simulink model "ACC_CC_model_4_15"  (R2018b)
settings: Solver=FixedStepAuto  StartTime=0.0  StopTime=20  RelTol=1e-3
InitFcn:
  | step=0.001;%时间步长
  | 
  | 
  | run parma2.m
libraries: simulink x2, Solver_SF x1, fuzblock x1
settings Model: Creator=Administrator  LastModifiedBy=61602
settings SFSimCC: SimUseLocalCustomCode=off
settings RTWCC: RTWUseLocalCustomCode=off

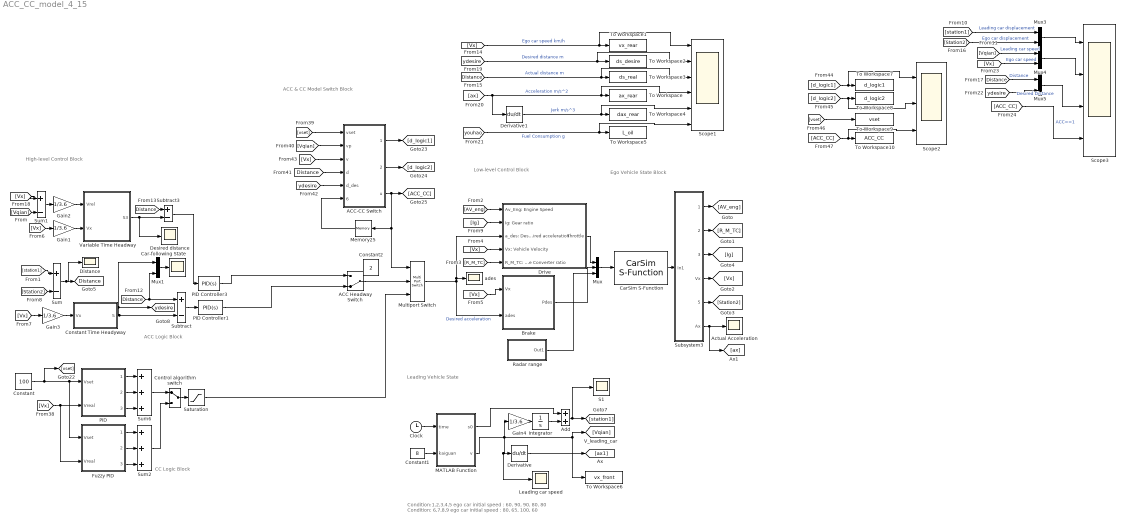
== system ACC_CC_model_4_15 ==
  note: Condition:1,2,3,4,5 ego car initial speed：60, 90, 90, 80, 80
      | Condition: 6,7,8,9   ego car initial speed：80, 65, 100, 60
  note: Leading Vehicle State
  note: ACC & CC Model
      | Switch Block
  note: High-level Control Block
  note: ACC Logic Block
  note: CC Logic Block
  note: Low-level
      | Control Block
  note: Ego Vehicle State
      | Block
  ACC Headway Switch : ManualSwitch  CurrentSetting=0
  ACC-CC Switch : MATLAB Function  TreatAsAtomicUnit=on
  Actual Acceleration : Scope
  Add : Sum
  Brake : Subsystem
  Car-following State : Scope
  "CarSim S-Function " : Solver_SF/CarSim S-Function  Priority=1  SIMFILE=simfile.sim
  Clock : Clock
  Constant : Constant  Value=100
  Constant Time Headyway : Subsystem
  Constant1 : Constant  Value=8
  Constant2 : Constant  Value=2
  Control algorithm switch : ManualSwitch
  Derivative : Derivative
  Derivative1 : Derivative
  "Desired distance " : Scope
  Distance : Scope
  Drive : Subsystem
  Fuzzy PID : Subsystem
  Gain{1..4} (4 alike) : Gain  Gain=1/3.6
  Integrator : Integrator
  Leading car speed : Scope
  MATLAB Function : MATLAB Function  TreatAsAtomicUnit=on
  Memory25 : Memory
  Multiport Switch : MultiPortSwitch  Inputs=2
  Mux : Mux  Inputs=3
  Mux{1,3..5} (4 alike) : Mux  Inputs=2
  PID : Subsystem
  PID Controller1 : simulink/Continuous/PID Controller  Controller=PID  Form=Parallel  TimeDomain=Continuous-time  SampleTime=-1  IntegratorMethod=Forward Euler  FilterMethod=Forward Euler  ControllerParametersSource=internal  P=4  I=0.01  D=2  UseFilter=on  N=100  TunerSelectOption=Transfer Function Based (PID Tuner App)  InitialConditionSource=internal  InitialConditionForIntegrator=0  InitialConditionForFilter=0  DifferentiatorICPrevScaledInput=0  ExternalReset=none  TrackingMode=off  Kt=1  LimitOutput=off  UpperSaturationLimit=inf  LowerSaturationLimit=-inf  LinearizeAsGain=on  AntiWindupMode=none  Kb=1  POutMin=[]  POutMax=[]  IOutMin=[]  IOutMax=[]  DOutMin=[]  DOutMax=[]  NOutMin=[]  NOutMax=[]  SumOutMin=[]  SumOutMax=[]  SaturationOutMin=[]  SaturationOutMax=[]  PParamMin=[]  PParamMax=[]  IParamMin=[]  IParamMax=[]  DParamMin=[]  DParamMax=[]  NParamMin=[]  NParamMax=[]  KbParamMin=[]  KbParamMax=[]  KtParamMin=[]  KtParamMax=[]  KbOutMin=[]  KbOutMax=[]  KtOutMin=[]  KtOutMax=[]  IntegratorOutMin=[]  IntegratorOutMax=[]  FilterOutMin=[]  FilterOutMax=[]  SumI1OutMin=[]  SumI1OutMax=[]  SumI2OutMin=[]  SumI2OutMax=[]  SumI3OutMin=[]  SumI3OutMax=[]  SumI4OutMin=[]  SumI4OutMax=[]  SumDOutMin=[]  SumDOutMax=[]  DifferentiatorOutMin=[]  DifferentiatorOutMax=[]  FilterDiffOutCoefMin=[]  FilterDiffOutCoefMax=[]  ReciprocalOutMin=[]  ReciprocalOutMax=[]  SumDenOutMin=[]  SumDenOutMax=[]  SumNumOutMin=[]  SumNumOutMax=[]  DivideOutMin=[]  DivideOutMax=[]  IntegratorContinuousStateAttributes=''  IntegratorStateMustResolveToSignalObject=off  IntegratorRTWStateStorageClass=Auto  FilterContinuousStateAttributes=''  FilterStateMustResolveToSignalObject=off  FilterRTWStateStorageClass=Auto  ParallelPVariant=InternalParameters  IdealPVariant=Disabled  IVariant=InternalParameters  DVariant=InternalParameters  IntegratorVariant=Continuous  SatVariant=Disabled  AWVariant=Passthrough  PCopyVariant=Disabled  TRVariant=Disabled  FdbkBlocksVariant=Forward  IdealPFdbkVariant=Disabled  SatFdbkVariant=Disabled  DerivativeFilterVariant=ContFilter  NVariant=InternalParameters  NCopyVariant=Disabled  FilterICVariant=InternalICsFilter  IntegratorICVariant=InternalICs  ExternalResetVariant=Disabled  TRSumVariant=Passthrough  SumFdbkVariant=Disabled  SumVariant=Sum_PID
  PID Controller3 : simulink/Continuous/PID Controller  Controller=PID  Form=Parallel  TimeDomain=Continuous-time  SampleTime=-1  IntegratorMethod=Forward Euler  FilterMethod=Forward Euler  ControllerParametersSource=internal  P=4  I=0.01  D=2  UseFilter=on  N=100  TunerSelectOption=Transfer Function Based (PID Tuner App)  InitialConditionSource=internal  InitialConditionForIntegrator=0  InitialConditionForFilter=0  DifferentiatorICPrevScaledInput=0  ExternalReset=none  TrackingMode=off  Kt=1  LimitOutput=off  UpperSaturationLimit=inf  LowerSaturationLimit=-inf  LinearizeAsGain=on  AntiWindupMode=none  Kb=1  POutMin=[]  POutMax=[]  IOutMin=[]  IOutMax=[]  DOutMin=[]  DOutMax=[]  NOutMin=[]  NOutMax=[]  SumOutMin=[]  SumOutMax=[]  SaturationOutMin=[]  SaturationOutMax=[]  PParamMin=[]  PParamMax=[]  IParamMin=[]  IParamMax=[]  DParamMin=[]  DParamMax=[]  NParamMin=[]  NParamMax=[]  KbParamMin=[]  KbParamMax=[]  KtParamMin=[]  KtParamMax=[]  KbOutMin=[]  KbOutMax=[]  KtOutMin=[]  KtOutMax=[]  IntegratorOutMin=[]  IntegratorOutMax=[]  FilterOutMin=[]  FilterOutMax=[]  SumI1OutMin=[]  SumI1OutMax=[]  SumI2OutMin=[]  SumI2OutMax=[]  SumI3OutMin=[]  SumI3OutMax=[]  SumI4OutMin=[]  SumI4OutMax=[]  SumDOutMin=[]  SumDOutMax=[]  DifferentiatorOutMin=[]  DifferentiatorOutMax=[]  FilterDiffOutCoefMin=[]  FilterDiffOutCoefMax=[]  ReciprocalOutMin=[]  ReciprocalOutMax=[]  SumDenOutMin=[]  SumDenOutMax=[]  SumNumOutMin=[]  SumNumOutMax=[]  DivideOutMin=[]  DivideOutMax=[]  IntegratorContinuousStateAttributes=''  IntegratorStateMustResolveToSignalObject=off  IntegratorRTWStateStorageClass=Auto  FilterContinuousStateAttributes=''  FilterStateMustResolveToSignalObject=off  FilterRTWStateStorageClass=Auto  ParallelPVariant=InternalParameters  IdealPVariant=Disabled  IVariant=InternalParameters  DVariant=InternalParameters  IntegratorVariant=Continuous  SatVariant=Disabled  AWVariant=Passthrough  PCopyVariant=Disabled  TRVariant=Disabled  FdbkBlocksVariant=Forward  IdealPFdbkVariant=Disabled  SatFdbkVariant=Disabled  DerivativeFilterVariant=ContFilter  NVariant=InternalParameters  NCopyVariant=Disabled  FilterICVariant=InternalICsFilter  IntegratorICVariant=InternalICs  ExternalResetVariant=Disabled  TRSumVariant=Passthrough  SumFdbkVariant=Disabled  SumVariant=Sum_PID
  Radar range : Subsystem
  S1 : Scope
  Saturation : Saturate  UpperLimit=2  LowerLimit=-2
  Scope1 : Scope  NumInputPorts=6
  Scope2 : Scope  NumInputPorts=3
  Scope3 : Scope  NumInputPorts=4
  Subsystem3 : Subsystem
  Subtract : Sum  Inputs=+-
  Subtract3 : Sum  Inputs=+-
  Sum : Sum  Inputs=+|-
  Sum1 : Sum  Inputs=+|-
  Sum2 : Sum  Inputs=+++
  Sum6 : Sum  Inputs=+++
  To Workspace : ToWorkspace  VariableName=ax_rear  SampleTime=-1
  To Workspace1 : ToWorkspace  VariableName=vx_rear  SampleTime=-1
  To Workspace10 : ToWorkspace  VariableName=ACC_CC  SampleTime=-1
  To Workspace2 : ToWorkspace  VariableName=ds_desire  SampleTime=-1
  To Workspace3 : ToWorkspace  VariableName=ds_real  SampleTime=-1
  To Workspace4 : ToWorkspace  VariableName=dax_rear  SampleTime=-1
  To Workspace5 : ToWorkspace  VariableName=L_oil  SampleTime=-1
  To Workspace6 : ToWorkspace  VariableName=vx_front  SampleTime=-1
  To Workspace7 : ToWorkspace  VariableName=d_logic1  SampleTime=-1
  To Workspace8 : ToWorkspace  VariableName=d_logic2  SampleTime=-1
  To Workspace9 : ToWorkspace  VariableName=vset  SampleTime=-1
  Variable Time Headway : Subsystem
  ades : Scope
  tag scope: Distance=global, ydesire=global
  wires:
  Subtract/1 -> PID Controller1/1
  Gain1/1 -> Variable Time Headway/2(Vx)
  Constant Time Headyway/1(S) -> Mux1/1, [ydesire], Subtract/2
  Brake/1("Pdes ") -> Mux/2
  "CarSim S-Function "/1 -> Subsystem3/1(In1)
  Mux/1 -> "CarSim S-Function "/1
  Gain2/1 -> Variable Time Headway/1(Vrel)
  Subsystem3/6(Ax) -> [ax], Actual Acceleration/1
  Drive/1("Throttle ") -> Mux/1
  Add/1 -> S1/1, [station1]
  MATLAB Function/2(v) -> Leading car speed/1, Derivative/1, Gain4/1, To Workspace6/1, [Vqian]
  Derivative/1 -> [ax1]
  [Vqian] -> Sum1/2
  Sum1/1 -> Gain2/1
  [station1] -> Sum/1
  Variable Time Headway/1(S3) -> "Desired distance "/1, Subtract3/2
  Subtract3/1 -> PID Controller3/1
  Subsystem3/1(AV_Eng) -> [AV_eng]
  [AV_eng] -> Drive/1(Av_Eng: Engine Speed)
  Subsystem3/2(R_M_TC) -> [R_M_TC]
  [R_M_TC] -> Drive/5(R_M_TC: Torque Converter ratio)
  Subsystem3/4(Vx) -> [Vx]
  [Vx] -> Brake/1(Vx)
  [Vx] -> Drive/4(Vx: Vehicle Velocity)
  [Vx] -> Gain1/1
  Subsystem3/5(station2) -> [Station2]
  [Station2] -> Sum/2
  Subsystem3/3(Rgear_Tr) -> [Ig]
  [Ig] -> Drive/2(Ig: Gear ratio)
  Sum/1 -> Distance/1, [Distance]
  [Distance] -> Mux1/2, Subtract/1
  [Distance] -> Subtract3/1
  PID Controller3/1 -> ACC Headway Switch/1
  Multiport Switch/1 -> Brake/2(ades), Drive/3(a_des: Desired acceleration), ades/1  "Desired acceleration"
  [Vx] -> Gain3/1
  Gain3/1 -> Constant Time Headyway/1(Vx)
  Mux1/1 -> Car-following State/1
  PID Controller1/1 -> ACC Headway Switch/2
  [Vx] -> Sum1/1
  PID/3(3) -> Sum6/3
  Constant/1 -> [vset], Fuzzy PID/1(Vset), PID/1(Vset)
  PID/2(2) -> Sum6/2
  PID/1(1) -> Sum6/1
  Control algorithm switch/1 -> Saturation/1
  Clock/1 -> MATLAB Function/1(time)
  [ydesire] -> Scope1/2, To Workspace2/1  "Desired distance m"
  [Vx] -> Scope1/1, To Workspace1/1  "Ego car speed km/h"
  [Distance] -> Scope1/3, To Workspace3/1  "Actual distance m"
  [ax] -> Derivative1/1, Scope1/4, To Workspace/1  "Acceleration m/s^2"
  Derivative1/1 -> Scope1/5, To Workspace4/1  "Jerk m/s^3"
  [youhao] -> Scope1/6, To Workspace5/1  "Fuel Consumption g"
  Gain4/1 -> Integrator/1
  Integrator/1 -> Add/2
  MATLAB Function/1(s0) -> Add/1
  Constant1/1 -> MATLAB Function/2(kaiguan)
  ACC-CC Switch/3(u) -> [ACC_CC], Multiport Switch/1, Memory25/1
  [Vx] -> Fuzzy PID/2(Vreal), PID/2(Vreal)
  [vset] -> ACC-CC Switch/1(vset)
  [Vqian] -> ACC-CC Switch/2(vp)
  [Distance] -> ACC-CC Switch/4(d)
  [ydesire] -> ACC-CC Switch/5(d_des)
  [Vx] -> ACC-CC Switch/3(v)
  Memory25/1 -> ACC-CC Switch/6(lastmodel)
  ACC-CC Switch/1(d_logic1) -> [d_logic1]
  ACC-CC Switch/2(d_logic2) -> [d_logic2]
  [d_logic1] -> Scope2/1, To Workspace7/1
  [d_logic2] -> Scope2/2, To Workspace8/1
  [vset] -> To Workspace9/1
  [ACC_CC] -> Scope2/3, To Workspace10/1
  ACC Headway Switch/1 -> Multiport Switch/2
  Saturation/1 -> Multiport Switch/3
  Fuzzy PID/1(1) -> Sum2/1
  Fuzzy PID/2(2) -> Sum2/2
  Fuzzy PID/3(3) -> Sum2/3
  Sum6/1 -> Control algorithm switch/1
  Sum2/1 -> Control algorithm switch/2
  Radar range/1(Out1) -> Mux/3
  Mux3/1 -> Scope3/1
  [station1] -> Mux3/1  "Leading car displacement"
  [Station2] -> Mux3/2  "Ego car displacement"
  Mux4/1 -> Scope3/2
  [Vqian] -> Mux4/1  "Leading car speed"
  [Vx] -> Mux4/2  "Ego car speed"
  Mux5/1 -> Scope3/3
  [Distance] -> Mux5/1  "Distance"
  [ydesire] -> Mux5/2  "Desired Distance"
  [ACC_CC] -> Scope3/4  "ACC==1"

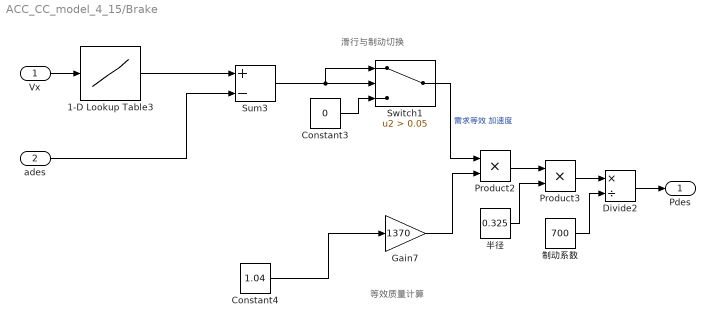
== system ACC_CC_model_4_15/Brake ==
  note: 滑行与制动切换
  note: 等效质量计算
  Vx : Inport
  ades : Inport  Port=2
  1-D Lookup Table3 : Lookup_n-D  NumberOfTableDimensions=1  BreakpointsForDimension1=[31.161 42.544 43.731 60.431 61.327 74.254 75.115 101.91 150.66]  Table=[-0.23293 -0.31787 -0.19431 -0.2768 -0.193 -0.24877 -0.21234 -0.33737 -0.63461]  InterpMethod=Cubic spline  InternalRulePriority=Speed  RndMeth=Simplest  InputSameDT=on
  Constant3 : Constant  Value=0
  Constant4 : Constant  Value=1.04
  Divide2 : Product  Inputs=*/
  Gain7 : Gain  Gain=1370
  Product2 : Product
  Product3 : Product
  Sum3 : Sum  Inputs=+|-
  Switch1 : Switch  Criteria=u2 > Threshold  Threshold=0.05
  制动系数 : Constant  Value=700
  半径 : Constant  Value=0.325
  "Pdes " : Outport
  wires:
  Vx/1 -> 1-D Lookup Table3/1
  1-D Lookup Table3/1 -> Sum3/1
  Sum3/1 -> Switch1/2, Switch1/1
  Constant3/1 -> Switch1/3
  ades/1 -> Sum3/2
  Switch1/1 -> Product2/1  "需求等效 加速度"
  Constant4/1 -> Gain7/1
  Gain7/1 -> Product2/2
  Product2/1 -> Product3/1
  半径/1 -> Product3/2
  Product3/1 -> Divide2/1
  制动系数/1 -> Divide2/2
  Divide2/1 -> "Pdes "/1

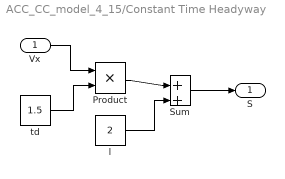
== system ACC_CC_model_4_15/Constant Time Headyway ==
  Vx : Inport
  Product : Product
  Sum : Sum  Inputs=+|+
  l : Constant  Value=2
  td : Constant  Value=1.5
  S : Outport
  wires:
  td/1 -> Product/2
  Vx/1 -> Product/1
  Product/1 -> Sum/1
  Sum/1 -> S/1
  l/1 -> Sum/2

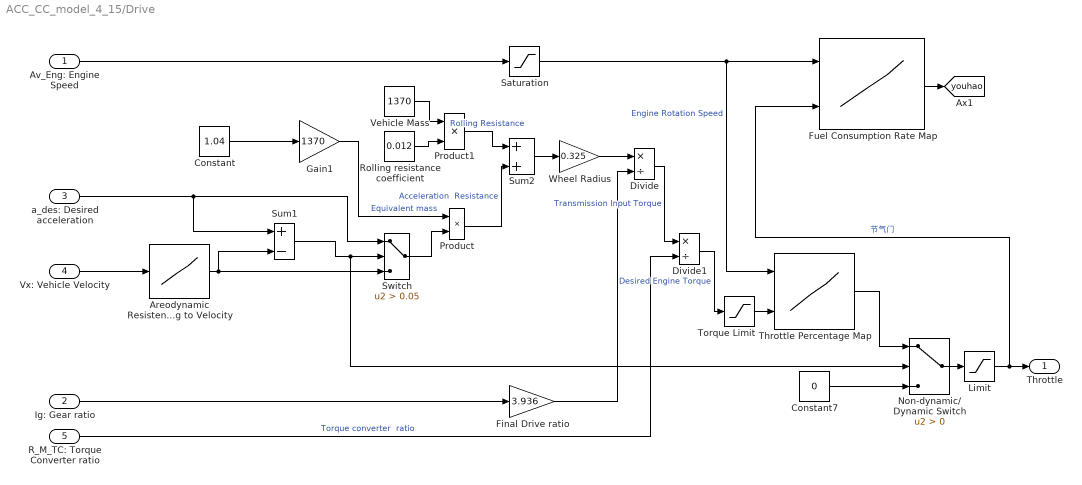
== system ACC_CC_model_4_15/Drive ==
  Av_Eng: Engine Speed : Inport
  Ig: Gear ratio : Inport  Port=2
  a_des: Desired acceleration : Inport  Port=3
  Vx: Vehicle Velocity : Inport  Port=4
  R_M_TC: Torque Converter ratio : Inport  Port=5
  Areodynamic Resistence corresponding to Velocity : Lookup_n-D  NumberOfTableDimensions=1  BreakpointsForDimension1=[31.161 42.544 43.731 60.431 61.327 74.254 75.115 101.91 150.66]  Table=[-0.23293 -0.31787 -0.19431 -0.2768 -0.193 -0.24877 -0.21234 -0.33737 -0.63461]  InterpMethod=Cubic spline  ExtrapMethod=Cubic spline  InternalRulePriority=Speed  RndMeth=Simplest  InputSameDT=on
  Constant : Constant  Value=1.04
  Constant7 : Constant  Value=0
  Divide : Product  Inputs=*/
  Divide1 : Product  Inputs=*/
  Final Drive ratio : Gain  Gain=3.936
  Fuel Consumption Rate Map : Lookup_n-D  BreakpointsSpecification=Even spacing  BreakpointsForDimension1=[0 600 800 1000 1200 1400 1600 1800 2000 2200 2400 2600 2800 3200 3600 4000 4400 4800 5200 5600 5800]  BreakpointsForDimension2=[0 0.04 0.08 0.12 0.16 0.2 0.24 0.28 0.32 0.36 0.4 0.44 0.48 0.52 0.56 0.6 0.64 0.68 0.72 0.76 0.8 0.84 0.88 0.92 0.96 1]  BreakpointsForDimension1FirstPoint=0  BreakpointsForDimension2FirstPoint=0  BreakpointsForDimension1Spacing=200  BreakpointsForDimension2Spacing=0.04  Table="[8.00E-05\t0.0002\t0.0003\t0.00032\t0.00034\t0.00037\t0.00039\t0.00041\t0.00043\t0.00046\t0.00048\t0.0005\t0.00052\t0.00055\t0.00057\t0.00059\t0.00061\t0.00064\t0.00066\t0.00068\t0.0007\t0.00073\t0.00075\t0.00077\t0.00079\t0.00082;0.00013\t0.0002\t0.0004\t0.00059\t0.00071\t0.0008\t0.00083\t0.00085\t0.00086\t0.00087\t0.00088\t0.00089\t0.0009\t0.00091\t0.00092\t0.00093\t0.00094\t0.00096\t0.00097\t0.00098\t0.00099\t0.001\t0.00101\t0.00102\t0.00103\t0.00104;0.00016\t0.0002\t0.00039\t0.00062\t0.00079\t0.00091\t0.00099\t0.00104\t0.00107\t0.00108\t0.00109\t0.00111\t0.00112\t0.00113\t0.00114\t0.00115\t0.00117\t0.00118\t0.00119\t0.0012\t0.00121\t0.00123\t0.00124\t0.00125\t0.00126\t0.00127;0.00016\t0.00021\t0.00039\t0.00064\t0.00088\t0.00104\t0.00114\t0.00123\t0.00128\t0.00131\t0.00133\t0.00134\t0.00135\t0.00137\t0.00138\t0.0014\t0.00141\t0.00142\t0.00144\t0.00145\t0.00147\t0.00148\t0.00149\t0.00151\t0.00152\t0.00154;0.00017\t0.00023\t0.00039\t0.00066\t0.00091\t0.00113\t0.0013\t0.0014\t0.00148\t0.00153\t0.00156\t0.00158\t0.0016\t0.00161\t0.00163\t0.00165\t0.00167\t0.00168\t0.0017\t0.00172\t0.00174\t0.00175\t0.00177\t0.00179\t0.00181\t0.00182;0.0002\t0.00026\t0.0004\t0.00066\t0.00095\t0.00119\t0.00139\t0.00154\t0.00164\t0.00173\t0.00178\t0.00181\t0.00183\t0.00184\t0.00186\t0.00188\t0.0019\t0.00192\t0.00194\t0.00195\t0.00197\t0.00199\t0.00201\t0.00203\t0.00205\t0.00207;0.00021\t0.00028\t0.00039\t0.00067\t0.00095\t0.00124\t0.00147\t0.00166\t0.00178\t0.00189\t0.00195\t0.002\t0.00203\t0.00206\t0.00209\t0.00212\t0.00215\t0.00218\t0.00222\t0.00225\t0.00228\t0.00231\t0.00234\t0.00237\t0.0024\t0.00243;0.00023\t0.0003\t0.00038\t0.00065\t0.00096\t0.00129\t0.00156\t0.00178\t0.00195\t0.00207\t0.00215\t0.00221\t0.00227\t0.00231\t0.00234\t0.00238\t0.00241\t0.00245\t0.00249\t0.00252\t0.00256\t0.00259\t0.00263\t0.00267\t0.0027\t0.00274;0.00025\t0.00033\t0.00041\t0.00065\t0.00098\t0.0013\t0.00162\t0.00189\t0.00212\t0.00226\t0.00239\t0.00246\t0.00252\t0.00257\t0.00261\t0.00264\t0.00268\t0.00272\t0.00275\t0.00279\t0.00282\t0.00286\t0.0029\t0.00293\t0.00297\t0.003;0.00027\t0.00036\t0.00044\t0.00065\t0.00095\t0.00133\t0.00168\t0.00199\t0.00223\t0.0024\t0.00255\t0.00265\t0.00272\t0.00278\t0.00284\t0.0029\t0.00296\t0.00302\t0.00308\t0.00314\t0.00319\t0.00325\t0.00331\t0.00337\t0.00343\t0.00349;0.0003\t0.000375\t0.00045\t0.00065\t0.00096\t0.001335\t0.00171\t0.00203\t0.00231\t0.002525\t0.002675\t0.002805\t0.002895\t0.002955\t0.00302\t0.00308\t0.003135\t0.00319\t0.00325\t0.003305\t0.003355\t0.00341\t0.00347\t0.003525\t0.00358\t0.00364;0.00033\t0.00039\t0.00046\t0.00065\t0.00097\t0.00134\t0.00174\t0.00207\t0.00239\t0.00265\t0.0028\t0.00296\t0.00307\t0.00313\t0.0032\t0.00326\t0.00331\t0.00336\t0.00342\t0.00347\t0.00352\t0.00357\t0.00363\t0.00368\t0.00373\t0.00379;0.000355\t0.00042\t0.000495\t0.000645\t0.00097\t0.00135\t0.001745\t0.002115\t0.002475\t0.00276\t0.00295\t0.00311\t0.00325\t0.00339\t0.00354\t0.00368\t0.003775\t0.003805\t0.003845\t0.00388\t0.00391\t0.003945\t0.003985\t0.004015\t0.00405\t0.00409;0.00038\t0.00045\t0.00053\t0.00064\t0.00097\t0.00136\t0.00175\t0.00216\t0.00256\t0.00287\t0.0031\t0.00326\t0.00343\t0.00365\t0.00388\t0.0041\t0.00424\t0.00425\t0.00427\t0.00429\t0.0043\t0.00432\t0.00434\t0.00435\t0.00437\t0.00439;0.000405\t0.000485\t0.00057\t0.00067\t0.00096\t0.001365\t0.00177\t0.002185\t0.00264\t0.00301\t0.003285\t0.00355\t0.00383\t0.00414\t0.004375\t0.004525\t0.00463\t0.00467\t0.0047\t0.004715\t0.00473\t0.004745\t0.004765\t0.004775\t0.00479\t0.00481;0.00043\t0.00052\t0.00061\t0.0007\t0.00095\t0.00137\t0.00179\t0.00221\t0.00272\t0.00315\t0.00347\t0.00384\t0.00423\t0.00463\t0.00487\t0.00495\t0.00502\t0.00509\t0.00513\t0.00514\t0.00516\t0.00517\t0.00519\t0.0052\t0.00521\t0.00523;0.00045\t0.000555\t0.00072\t0.00094\t0.001285\t0.001735\t0.00219\t0.00269\t0.003195\t0.00359\t0.003915\t0.004355\t0.0048\t0.00525\t0.00545\t0.005515\t0.00558\t0.005645\t0.005685\t0.005695\t0.00571\t0.00572\t0.00574\t0.00575\t0.00576\t0.00578;0.00047\t0.00059\t0.00083\t0.00118\t0.00162\t0.0021\t0.00259\t0.00317\t0.00367\t0.00403\t0.00436\t0.00487\t0.00537\t0.00587\t0.00603\t0.00608\t0.00614\t0.0062\t0.00624\t0.00625\t0.00626\t0.00627\t0.00629\t0.0063\t0.00631\t0.00633;0.00049\t0.000615\t0.00084\t0.0012\t0.001635\t0.00214\t0.002645\t0.00325\t0.003795\t0.00423\t0.004565\t0.005005\t0.005525\t0.00604\t0.00639\t0.006555\t0.006615\t0.006675\t0.006725\t0.006755\t0.006785\t0.006795\t0.00681\t0.006825\t0.006835\t0.006855;0.00051\t0.00064\t0.00085\t0.00122\t0.00165\t0.00218\t0.0027\t0.00333\t0.00392\t0.00443\t0.00477\t0.00514\t0.00568\t0.00621\t0.00675\t0.00703\t0.00709\t0.00715\t0.00721\t0.00726\t0.00731\t0.00732\t0.00733\t0.00735\t0.00736\t0.00738;0.000515\t0.00069\t0.0009\t0.001215\t0.00166\t0.00218\t0.00271\t0.003345\t0.00398\t0.00451\t0.005075\t0.00577\t0.006345\t0.00673\t0.007125\t0.007385\t0.00751\t0.00757\t0.00763\t0.007685\t0.00774\t0.00777\t0.007805\t0.00782\t0.00783\t0.007845;0.00052\t0.00074\t0.00095\t0.00121\t0.00167\t0.00218\t0.00272\t0.00336\t0.00404\t0.00459\t0.00538\t0.0064\t0.00701\t0.00725\t0.0075\t0.00774\t0.00793\t0.00799\t0.00805\t0.00811\t0.00817\t0.00822\t0.00828\t0.00829\t0.0083\t0.00831;0.000555\t0.00076\t0.000965\t0.00119\t0.001655\t0.00217\t0.00272\t0.00338\t0.00407\t0.00482\t0.005855\t0.00665\t0.00724\t0.00752\t0.007785\t0.008045\t0.00828\t0.008395\t0.008455\t0.00851\t0.00857\t0.008625\t0.008685\t0.008715\t0.00875\t0.008785;0.00059\t0.00078\t0.00098\t0.00117\t0.00164\t0.00216\t0.00272\t0.0034\t0.0041\t0.00505\t0.00633\t0.0069\t0.00747\t0.00779\t0.00807\t0.00835\t0.00863\t0.0088\t0.00886\t0.00891\t0.00897\t0.00903\t0.00909\t0.00914\t0.0092\t0.00926;0.00062\t0.000805\t0.00099\t0.00118\t0.00162\t0.00214\t0.002725\t0.00348\t0.00436\t0.00528\t0.006355\t0.00697\t0.007545\t0.00791\t0.008185\t0.00846\t0.00874\t0.00896\t0.009055\t0.00911\t0.00917\t0.00923\t0.00929\t0.009345\t0.009405\t0.009465;0.00065\t0.00083\t0.001\t0.00119\t0.0016\t0.00212\t0.00273\t0.00356\t0.00462\t0.00551\t0.00638\t0.00704\t0.00762\t0.00803\t0.0083\t0.00857\t0.00885\t0.00912\t0.00925\t0.00931\t0.00937\t0.00943\t0.00949\t0.00955\t0.00961\t0.00967;0.00076\t0.0009\t0.00103\t0.00119\t0.00162\t0.00211\t0.00271\t0.00357\t0.0046\t0.00548\t0.00642\t0.00712\t0.00772\t0.00816\t0.00841\t0.00867\t0.00892\t0.00918\t0.0093\t0.00935\t0.0094\t0.00945\t0.00951\t0.00956\t0.00961\t0.00966]"  InternalRulePriority=Speed  RndMeth=Simplest  InputSameDT=on
  Gain1 : Gain  Gain=1370
  Limit : Saturate  UpperLimit=1  LowerLimit=0
  Non-dynamic/ Dynamic Switch : Switch  Criteria=u2 > Threshold  ZeroCross=off
  Product : Product
  Product1 : Product
  Rolling resistance coefficient : Constant  Value=0.012
  Saturation : Saturate  UpperLimit=6400  LowerLimit=0
  Sum1 : Sum  Inputs=+|-
  Sum2 : Sum
  Switch : Switch  Criteria=u2 > Threshold  Threshold=0.05  ZeroCross=off
  Throttle Percentage Map : Lookup_n-D  BreakpointsForDimension1=[0:200:6400]  BreakpointsForDimension2=[-80:20:400]  BreakpointsForDimension1FirstPoint=0  BreakpointsForDimension2FirstPoint=-80  BreakpointsForDimension1Spacing=200  BreakpointsForDimension2Spacing=20  Table="[0\t0\t0\t0\t0\t0\t0\t0\t0\t0\t0\t0\t0\t0\t0\t0\t0\t0\t0\t0\t0\t0\t0\t0\t0;0\t0\t0\t0\t0.00384203232361968\t0.00984257347407071\t0.0220398619570969\t0.0431381611163926\t0.0738017975356030\t0.110363332239170\t0.144256444326208\t0.164816882208714\t1\t1\t1\t1\t1\t1\t1\t1\t1\t0\t0\t0\t0;0\t0\t0\t0\t0.00233552878082050\t0.00619500499883992\t0.0144268956425663\t0.0294970721851443\t0.0529492390587595\t0.0834478836501531\t0.115463766954485\t0.140265514400698\t0.149599756648231\t0.140379561408988\t0.314838987863483\t1\t1\t1\t1\t1\t1\t1\t1\t1\t1;0\t0\t0\t0\t0.00269204644658483\t0.00655304149978634\t0.0142777145059634\t0.0278438877733882\t0.0486022596522765\t0.0759343803923640\t0.106188100327027\t0.132913365538591\t0.148907600349805\t0.149353518918563\t0.165691002544961\t0.443199346537509\t1\t1\t1\t0.0148015365144000\t0.00683120221226242\t0.00282191547531947\t0.00104338903135025\t0\t0;0\t0\t0\t0\t0.00316570810890816\t0.00743009581670684\t0.0156716784490837\t0.0297053150178035\t0.0505999822639421\t0.0774576147578403\t0.106555393386647\t0.131730539313129\t0.146412350396264\t0.148433510738055\t0.164082047248146\t0.287461695026555\t0.776435129008011\t1\t1\t1\t1\t1\t0.855344896028421\t0\t0;0.00156972662513287\t0.00292440315653881\t0.00521076920904484\t0\t0.0144740218296977\t0.0225640910928387\t0.0336445013564358\t0.0479845390368760\t0.0654692226693815\t0.0854804699717945\t0.106896491655099\t0.128321803338099\t0.148744855695550\t0.169069746657954\t0.195663523839765\t0.248850107320476\t0.383630461391210\t1\t1\t1\t1\t1\t1\t1\t1;0.00333772918734807\t0.00556793519844545\t0.00897138921617320\t0.0139620013536888\t0.0209873740927971\t0.0304712999653783\t0.0427313203239578\t0.0578794095739592\t0.0757223917941103\t0.0956856926738540\t0.116786364156857\t0.137676500902228\t0.156769917608745\t0.172704407828818\t0.190657800177763\t0.253117967669876\t0.345750076583537\t0.527683716791911\t1\t1\t1\t1\t0.324019751652870\t0.0661343442546140\t0.0496456670611000;0.00842938180192665\t0.0119379976727277\t0.0165972700848599\t0.0226522444373971\t0.0303497574277404\t0.0399179854909284\t0.0515408307577786\t0.0653286403635119\t0.0812877741322988\t0.0992924553748172\t0.119062960175288\t0.140154326369480\t0.161959390844382\t0.183786332740461\t0.208563512857288\t0.268671868208096\t0.347245115663011\t0.468148998702986\t1\t1\t1\t1\t1\t0.234534637403868\t0.217075267193582;0.00619741338574470\t0.00878361031910808\t0.0122867271926932\t0.0169628933569427\t0.0231134198821825\t0.0310834379029089\t0.0412566960616756\t0.0540456078109618\t0.0698758213850285\t0.0891649165686454\t0.112295318160444\t0.139582140263373\t0.171237396985538\t0.207332766445188\t0.247763850941385\t0.292254057085642\t0.343714301556105\t0.458144516741113\t0.890742933740108\t1\t1\t1\t1\t1\t1;0.00957767623630743\t0.0131188124891817\t0.0177530394518587\t0.0237353004082760\t0.0313516619998816\t0.0409138383586234\t0.0527501504567145\t0.0671925311576744\t0.0845594444667060\t0.105134938005879\t0.129144480351401\t0.156728814622521\t0.187919064393499\t0.222633113258974\t0.260840999456184\t0.303741390402770\t0.359217235661181\t0.458844921210738\t0.704450197768986\t1\t1\t1\t1\t1\t1;0.00999208439807737\t0.0139365359277347\t0.0191575884022884\t0.0259545851894262\t0.0346556940430014\t0.0456060399950533\t0.0591503585100480\t0.0756100722667621\t0.0952553066701650\t0.118273094676493\t0.144733811415315\t0.174558654188138\t0.207492325710677\t0.243097548860487\t0.280913227903114\t0.321694504502648\t0.373036414261962\t0.462584154163058\t0.645364008518645\t1\t1\t1\t1\t1\t1;0.0183965822224753\t0.0231535011658833\t0.0289998454240426\t0.0361471597043883\t0.0448386116510726\t0.0553515287633074\t0.0679996328295962\t0.0831348273800394\t0.101148376214565\t0.122471296470050\t0.147573779301476\t0.176963446513935\t0.211182253856597\t0.250801862650283\t0.296417327484778\t0.348639309948997\t0.408102014083543\t0.476231549167063\t0.583679054008124\t1\t1\t1\t1\t1\t1;0.00750164816735129\t0.0118958635783470\t0.0182879757097919\t0.0272563051726700\t0.0393824897819206\t0.0551672828234899\t0.0749236907300999\t0.0986628029405359\t0.125998589994764\t0.156108487254717\t0.187794870222566\t0.219112637863578\t0.250693298401737\t0.280532250949658\t0.310645255998005\t0.345051472732309\t0.391093453834695\t0.459609355163595\t0.564129276786969\t0.779583040338104\t1\t1\t1\t1\t1;0.0128310984809411\t0.0183783846673057\t0.0258118544185065\t0.0355467129742611\t0.0480007539242631\t0.0635572416292176\t0.0825183230105414\t0.105051949659107\t0.131137292174967\t0.160515394193700\t0.192652977018350\t0.226728093739513\t0.261651760288463\t0.296179876125557\t0.329346110575638\t0.361853055493373\t0.399038746999790\t0.453224626857502\t0.537525023193696\t0.656645690842970\t1\t1\t1\t1\t1;0.0247011121205898\t0.0317182638764303\t0.0403477295707015\t0.0508446880802143\t0.0634729767142210\t0.0784962549909302\t0.0961669408877947\t0.116713060543584\t0.140323337869647\t0.167131052657082\t0.197197399911042\t0.230495273276693\t0.266894570784037\t0.306150417619811\t0.347897274513490\t0.391663085274014\t0.436994592539312\t0.484285897291605\t0.539988960778002\t0.647902508602608\t1\t1\t1\t1\t1;0.00945454034963292\t0.0154749746931625\t0.0244119920347076\t0.0370916569053526\t0.0542484076650609\t0.0763339737226356\t0.103307387668274\t0.134470524934672\t0.168434387128764\t0.203296327963929\t0.237064438892021\t0.268281881129027\t0.296700700274079\t0.323770951611925\t0.352693915666079\t0.387870972549757\t0.433759113469211\t0.493374293069948\t0.567127733597060\t0.661541093732134\t0.987767242826757\t1\t1\t1\t1;0.00788947907416780\t0.0140737622591682\t0.0237835378253853\t0.0380899419524234\t0.0578431290248628\t0.0833596849828568\t0.114143714199600\t0.148774862455414\t0.185083227076750\t0.220650826514244\t0.253548792988966\t0.283090701486545\t0.310321430898121\t0.338011501183713\t0.370081392882042\t0.410578464538603\t0.462487583760790\t0.526738859478572\t0.602863553596186\t0.719375327298920\t1\t1\t1\t1\t1;0.00760157702493746\t0.0141354316304181\t0.0247569030989165\t0.0407855798120631\t0.0631816321102009\t0.0920843068201473\t0.126459377868593\t0.164085910805724\t0.202032172516139\t0.237563646161062\t0.269182110200302\t0.297358539641943\t0.324600782015269\t0.354772226899832\t0.391905629672254\t0.438957290455749\t0.496931671308596\t0.564854750166630\t0.646458197505932\t0.846713860317663\t1\t1\t1\t1\t1;0.0283613669950916\t0.0379391697994668\t0.0500058933165453\t0.0649422394898845\t0.0831009596301597\t0.104774967298857\t0.130161270058885\t0.159323145243383\t0.192153871285956\t0.228346103014216\t0.267371739224846\t0.308478547453642\t0.350714422369269\t0.393006333189035\t0.434375081061274\t0.474539409846220\t0.515694139207642\t0.567838348157797\t0.664681614423615\t0.910439138890854\t1\t1\t1\t1\t1;0.0290493539086180\t0.0393924148495188\t0.0525272564685800\t0.0688736102176339\t0.0888008398349195\t0.112584234075123\t0.140357237633617\t0.172063944372956\t0.207417523764615\t0.245871447767687\t0.286611758824519\t0.328581463357760\t0.370556111346543\t0.411312122894393\t0.449989613441090\t0.486905369742722\t0.525452708442786\t0.576646684590168\t0.670060842780561\t0.880007746167966\t1\t1\t1\t1\t1;0.0309923261101243\t0.0421523562621871\t0.0563345081509432\t0.0739796253265510\t0.0954629221108354\t0.121043734584308\t0.150811671839846\t0.184634480435921\t0.222114225251569\t0.262559139232789\t0.304978748833802\t0.348110477759937\t0.390489946750649\t0.430594107207538\t0.467144068496533\t0.499833404320824\t0.531316998953113\t0.585390900116497\t0.710314942976216\t0.894002710663273\t1\t1\t1\t1\t1;0.0296427154578126\t0.0416053478631931\t0.0571206043808213\t0.0767101183318286\t0.100770850632798\t0.129494089194201\t0.162785307190093\t0.200198440344337\t0.240900957504260\t0.283687687745043\t0.327062085729746\t0.369404985550394\t0.409256193008772\t0.445749337034703\t0.479274873980009\t0.512515557123877\t0.552128289885678\t0.611577727791069\t0.716029964178593\t0.910906473332351\t1\t1\t1\t1\t1;0.0301554024019646\t0.0430534606105860\t0.0599480352123431\t0.0814101228698585\t0.107829507476908\t0.139309962095908\t0.175573248724695\t0.215893497851702\t0.259086027789001\t0.303573880871192\t0.347551541629300\t0.389260177242258\t0.427385741371435\t0.461595554207361\t0.493247192827834\t0.526343827572268\t0.568882497522438\t0.634859369532335\t0.747377774610794\t0.943580162911627\t1\t1\t1\t1\t1;0.0125032729694962\t0.0246376160831942\t0.0449596989781896\t0.0754048116443178\t0.115871802969058\t0.163296335024811\t0.212147491398923\t0.256628639650145\t0.293555126472507\t0.324052115976146\t0.352798897394081\t0.385228290174814\t0.424472597350162\t0.469849362584449\t0.517609595793018\t0.563814829537172\t0.609509569728732\t0.669377751025561\t0.784660372337494\t1\t1\t1\t1\t1\t1;0.0127495780251357\t0.0260081731965988\t0.0487016543474852\t0.0829175797789835\t0.127892363805553\t0.179018109006521\t0.229096975540885\t0.271824034662138\t0.305408398784526\t0.333584152540217\t0.363066129987766\t0.403866329035035\t0.443233269890985\t0.491568850430310\t0.539082371005249\t0.583237353682395\t0.630052710294601\t0.701639611312345\t0.844015447026297\t1\t1\t1\t1\t1\t1;0.00608618868980984\t0.0254473661875037\t0.0532087751384493\t0.0898860082000276\t0.134805119488799\t0.185692642245017\t0.238447326146682\t0.287364575374095\t0.326615110227074\t0.354663593433239\t0.380753080870682\t0.421352560792910\t0.476085840660330\t0.518760620361190\t0.543235459434839\t0.589832290320803\t0.678128842881687\t0.765062457558665\t0.963488180608847\t1\t1\t1\t1\t1\t1;0.00876785805968322\t0.0238251313184682\t0.0537280642808312\t0.100964317650311\t0.159480023697879\t0.215599624816592\t0.258252223667772\t0.289638072073616\t0.322655235808328\t0.365767198629499\t0.413329469905078\t0.454344268879181\t0.489071116120177\t0.527486901796047\t0.565635939844740\t0.623094094354984\t0.719918968626461\t0.802769286639991\t1\t1\t1\t0.333502624117370\t0.143700279711866\t0.0700870605635040\t0.0303560250773317;0.0180221114554173\t0.0366445153119691\t0.0672282489467882\t0.110833792743377\t0.164387944722412\t0.220798717697628\t0.272067286300606\t0.313833475282062\t0.347938127559408\t0.380753788094797\t0.418508508605864\t0.463241833814513\t0.512238262864337\t0.561133988518728\t0.609229831249888\t0.666087782915168\t0.760432031982381\t0.954663090457091\t1\t1\t1\t1\t1\t1\t1;0.0277244592487692\t0.0485425607617500\t0.0792051187265345\t0.120387529893084\t0.170634406364521\t0.226140452297834\t0.281566927874754\t0.331825626186510\t0.374144623952895\t0.409397966475087\t0.441938834984417\t0.477926115248508\t0.522908667971669\t0.579740349119965\t0.647601778677248\t0.722495671404500\t0.851546308766713\t1\t0.923918885404956\t0.954541755099682\t0.966605303799230\t0.954339487162867\t0.918420141247823\t0.861424875271402\t0.787431120596477;0.0406051076129493\t0.0624631068651615\t0.0920807525577163\t0.130102334314394\t0.176232478338755\t0.228958727887680\t0.285498551408681\t0.342084315635324\t0.394638375246951\t0.439801238452127\t0.476193326956020\t0.505761528193289\t0.536113695715409\t0.600001233874219\t0.693845693177591\t0.794252302123721\t1\t1\t1\t1\t1\t1\t1\t1\t1;0.0425620744297415\t0.0664740032187708\t0.0989945546926814\t0.140612693207398\t0.190587787865367\t0.246696348074992\t0.305351173832978\t0.362220914682351\t0.413350036181931\t0.456615203767090\t0.493213894586310\t0.528823032751117\t0.574116091447174\t0.644464952657905\t0.758818768287968\t0.937881910690616\t1\t1\t1\t1\t1\t1\t1\t1\t1;0.0165164052619005\t0.0592024593260268\t0.142421679629580\t0.234936054784750\t0.298947767843167\t0.354513382166282\t0.430031687210808\t0.504200653371543\t0.554242052629062\t0.667497191065714\t0.820859064802699\t1\t1\t1\t1\t1\t1\t1\t1\t1\t1\t1\t1\t1\t1;0.0259740616983990\t0.160221367511912\t0.403002085736409\t0.583795601127385\t1\t1\t1\t1\t1\t1\t1\t1\t1\t0.295558374328020\t0.0411102929246858\t0.00398207838392640\t0\t1\t1\t1\t1\t1\t1\t1\t1]"  InterpMethod=Cubic spline  ExtrapMethod=Clip  InternalRulePriority=Speed  RndMeth=Simplest  InputSameDT=on
  Torque Limit : Saturate  UpperLimit=400  LowerLimit=-80
  Vehicle Mass : Constant  Value=1370
  Wheel Radius : Gain  Gain=0.325
  "Throttle " : Outport
  tag scope: youhao=global
  wires:
  Final Drive ratio/1 -> Divide/2
  Sum2/1 -> Wheel Radius/1
  Wheel Radius/1 -> Divide/1
  Divide/1 -> Divide1/1  "Transmission Input Torque"
  R_M_TC: Torque Converter ratio/1 -> Divide1/2  "Torque converter  ratio"
  Divide1/1 -> Torque Limit/1  "Desired Engine Torque"
  Torque Limit/1 -> Throttle Percentage Map/2
  Saturation/1 -> Fuel Consumption Rate Map/1, Throttle Percentage Map/1  "Engine Rotation Speed"
  Throttle Percentage Map/1 -> Non-dynamic/ Dynamic Switch/1
  Constant7/1 -> Non-dynamic/ Dynamic Switch/3
  Non-dynamic/ Dynamic Switch/1 -> Limit/1
  Limit/1 -> "Throttle "/1, Fuel Consumption Rate Map/2  "节气门"
  Ig: Gear ratio/1 -> Final Drive ratio/1
  Constant/1 -> Gain1/1
  Gain1/1 -> Product/1  "Equivalent mass"
  a_des: Desired acceleration/1 -> Sum1/1, Switch/1
  Vx: Vehicle Velocity/1 -> Areodynamic Resistence corresponding to Velocity/1
  Sum1/1 -> Non-dynamic/ Dynamic Switch/2, Switch/2
  Switch/1 -> Product/2
  Vehicle Mass/1 -> Product1/1
  Rolling resistance coefficient/1 -> Product1/2
  Product/1 -> Sum2/2  "Acceleration  Resistance"
  Product1/1 -> Sum2/1  "Rolling Resistance"
  Av_Eng: Engine Speed/1 -> Saturation/1
  Areodynamic Resistence corresponding to Velocity/1 -> Switch/3, Sum1/2
  Fuel Consumption Rate Map/1 -> [youhao]

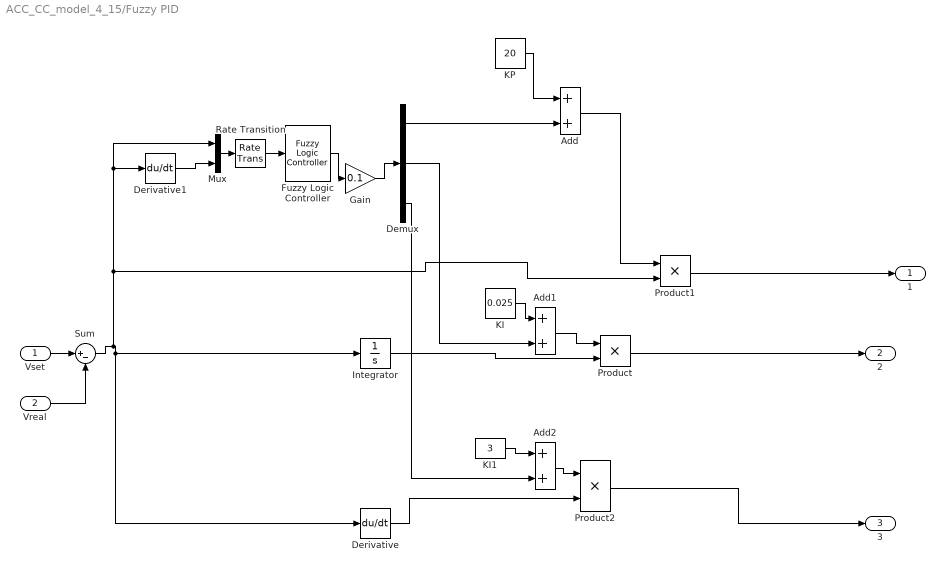
== system ACC_CC_model_4_15/Fuzzy PID ==
  Vset : Inport
  Vreal : Inport  Port=2
  Add : Sum
  Add1 : Sum
  Add2 : Sum
  Demux : Demux  Outputs=3
  Derivative : Derivative
  Derivative1 : Derivative
  Fuzzy Logic Controller : fuzblock/Fuzzy Logic  Controller  FIS='fuzzypid.fis'  OutputSampleNumber=101  DataType=double  FuzzifiedInputs=off  RuleFiringStrengths=off  RuleOutputs=off  AggregatedOutputs=off  SimulateUsing=Interpreted execution  OutOfRangeInputValueMessage=warning  NoRuleFiredMessage=warning  EmptyOutputFuzzySetMessage=warning
  Gain : Gain  Gain=0.1
  Integrator : Integrator
  KI : Constant  Value=0.025
  KI1 : Constant  Value=3
  KP : Constant  Value=20
  Mux : Mux  Inputs=2
  Product : Product
  Product1 : Product
  Product2 : Product
  Rate Transition : RateTransition  OutPortSampleTime=1
  Sum : Sum  Inputs=|+-
  1 : Outport
  2 : Outport  Port=2
  3 : Outport  Port=3
  wires:
  Vreal/1 -> Sum/2
  Sum/1 -> Derivative/1, Integrator/1, Product1/2, Mux/1, Derivative1/1
  Product2/1 -> 3/1
  Product/1 -> 2/1
  Derivative/1 -> Product2/2
  Product1/1 -> 1/1
  Integrator/1 -> Product/2
  Vset/1 -> Sum/1
  Derivative1/1 -> Mux/2
  Mux/1 -> Rate Transition/1
  Gain/1 -> Demux/1
  KP/1 -> Add/1
  Demux/1 -> Add/2
  KI/1 -> Add1/1
  Demux/2 -> Add1/2
  Add1/1 -> Product/1
  Add/1 -> Product1/1
  Add2/1 -> Product2/1
  KI1/1 -> Add2/1
  Demux/3 -> Add2/2
  Rate Transition/1 -> Fuzzy Logic Controller/1
  Fuzzy Logic Controller/1 -> Gain/1

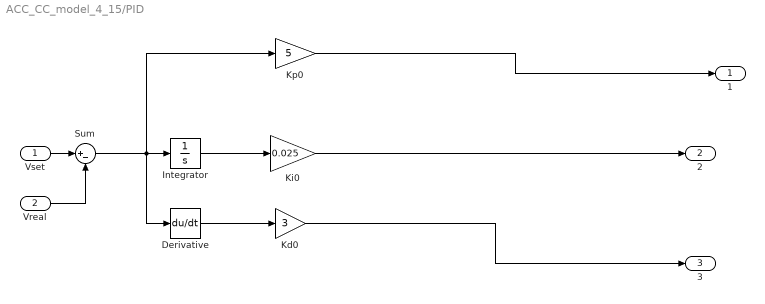
== system ACC_CC_model_4_15/PID ==
  Vset : Inport
  Vreal : Inport  Port=2
  Derivative : Derivative
  Integrator : Integrator
  Kd0 : Gain  Gain=3
  Ki0 : Gain  Gain=0.025
  Kp0 : Gain  Gain=5
  Sum : Sum  Inputs=|+-
  1 : Outport
  2 : Outport  Port=2
  3 : Outport  Port=3
  wires:
  Vset/1 -> Sum/1
  Integrator/1 -> Ki0/1
  Kp0/1 -> 1/1
  Derivative/1 -> Kd0/1
  Ki0/1 -> 2/1
  Kd0/1 -> 3/1
  Sum/1 -> Derivative/1, Integrator/1, Kp0/1
  Vreal/1 -> Sum/2

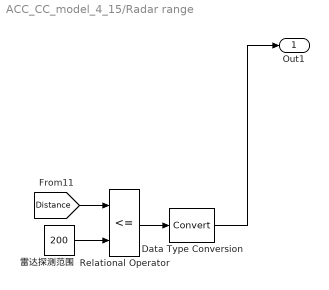
== system ACC_CC_model_4_15/Radar range ==
  Data Type Conversion : DataTypeConversion
  Relational Operator : RelationalOperator  Operator=<=  OutDataTypeStr=boolean  RndMeth=Simplest
  雷达探测范围 : Constant  Value=200
  Out1 : Outport
  wires:
  Data Type Conversion/1 -> Out1/1
  雷达探测范围/1 -> Relational Operator/2
  Relational Operator/1 -> Data Type Conversion/1
  [Distance] -> Relational Operator/1

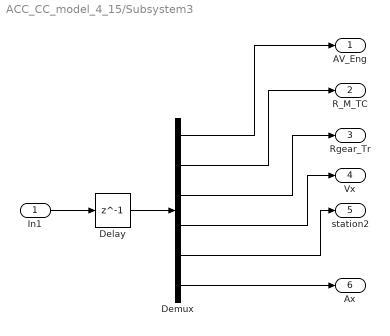
== system ACC_CC_model_4_15/Subsystem3 ==
  In1 : Inport
  Delay : Delay  DelayLength=1  InitialCondition=0
  Demux : Demux  Outputs=6
  AV_Eng : Outport
  R_M_TC : Outport  Port=2
  Rgear_Tr : Outport  Port=3
  Vx : Outport  Port=4
  station2 : Outport  Port=5
  Ax : Outport  Port=6
  wires:
  Demux/5 -> station2/1
  Demux/4 -> Vx/1
  Demux/3 -> Rgear_Tr/1
  Demux/2 -> R_M_TC/1
  Demux/1 -> AV_Eng/1
  In1/1 -> Delay/1
  Delay/1 -> Demux/1
  Demux/6 -> Ax/1

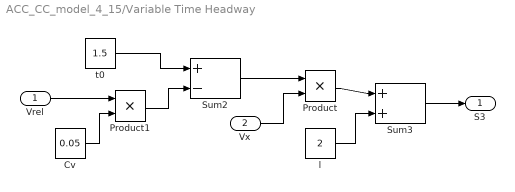
== system ACC_CC_model_4_15/Variable Time Headway ==
  Vrel : Inport
  Vx : Inport  Port=2
  Cv : Constant  Value=0.05
  Product : Product
  Product1 : Product
  Sum2 : Sum  Inputs=+|-
  Sum3 : Sum  Inputs=+|+
  l : Constant  Value=2
  t0 : Constant  Value=1.5
  S3 : Outport
  wires:
  Sum2/1 -> Product/1
  t0/1 -> Sum2/1
  Sum3/1 -> S3/1
  Product/1 -> Sum3/1
  Vx/1 -> Product/2
  Product1/1 -> Sum2/2
  l/1 -> Sum3/2
  Vrel/1 -> Product1/1
  Cv/1 -> Product1/2

== matlab function ACC_CC_model_4_15/MATLAB Function ==
  data: s0 output; time input; kaiguan input; v output
function [s0,v] = fcn(time,kaiguan)
td=1.5;   %s;
% switch=1~5 represents ACC operating conditions
% switch=6~9 represents ACC/CC switching conditions
 
switch kaiguan
    
    case 1  %% *****************************Leading vehicle accelerates

        %leading car accelerate condition
        %t<9s leading car constant speed at 60km/h
        %ego car keep 27m distance following
        %t=9s leading car accelerates with 1.6m/s^2 to 90km/h .
        if time<9
            v=60;
        else
            v=60+1.6*(time-9)*3.6;  %?1.6m/s^2
            if v>90
                v=90;
            end
        end
        s0=60/3.6*td+2;% leading car initial location
    case 2  %% *************************** Leading vehicle decelerates

        % t<9s leading car constant speed at 90km/h 
        % keep distance of 90/3.6*td+2 following
        % t=9s   leading car decelerates with -1.6m/s2 to 60km/h
        if time<9
            v=90;
        else
            v=90-1.6*(time-9)*3.6;  %-1.6m/s^2 
            if v<60
                v=60;
            end
        end
        s0=90/3.6*td+2;% leading car initial location
    case 3  %% ************************************* Steady following

        % leading car speed fluctuating at 90km/h 
        % figure
        % x=0:0.001:50;
        % y=sin(x*0.1)+sin(x*0.4)-sin(x*0.2)+sin(x*0.8)-sin(x*0.3);
        % plot(x,y)
        x=time;
        v=sin(x*0.1)+sin(x*0.4)-sin(x*0.2)+sin(x*0.8)-sin(x*0.3)+90;
        s0=90/3.6*td+2;% leading car initial location	    
    case 4  %% ***************************** Leading vehicle departs, following another leading vehicle

        % t<15s leading car constant speed at 80km/h 
        % ego car following with 45m distance
        % t=15s car in other line cuts in at 80km/h with 20m ahead
        % causing preestablished safety distance
        if time<15
            s0=80/3.6*td+2;%leading car initial location
            v=80;
        else
            s0=80/3.6*td+2-15.3333;% leading car initial location(a car cuts in)
            v=80;
        end
    case 5  %% ******************************************* Other vehicle cuts in the front

        % leading car constant speed at 80km/h ego car following with 35m 
        % t=10s leading car departs ego line
        % ACC trace another leading car 70m ahead at 80km/h
        if time<10
            v=80;
            s0=80/3.6*td+2;%leading car initial location
        else
            v=80;
            s0=80/3.6*td+2+35; %leading car initial location(leading car    departs)
        end
    case 6 %% ********************* Encounter leading vehicle (CC to ACC)

        % ego car CC 80km/h, leading car CC 60km/h 200m ahead
        % ego car switch from CC to ACC
       
        v=60;
        s0=200;%initial location 
    case 7 %% ******************************************* Leading vehicle departs, no another   leading vehicle. (ACC to CC)
        % t<9s leading car CC 65km/h 35m ahead, ego car following at 65km/h 
        % t=9s leading car departs and no car ahead then
        % ego car switch from ACC to CC at 80km/h
        if time<9
            v=65;
            s0=v/3.6*td+2; % leading car initial location
        else
            v=0;
            s0=10000;% leading car initial location (leading car departs)
        end
        
    case 8 %% ******************************************* Leading vehicle departs, encountering another leading vehicle (ACC-CC-ACC) )
        % t<9s leading car constant speed at 100km/h, ego car ACC following 9s 
        % t>9s leading car departs, 
        % ego car encounters another leading car 80m ahead at 70km/h
        % ego car switch from ACC to CC.
        if time<9
            v=100;
            s0=v/3.6*td+2;%leading car initial location
        else
            v=70;
            s0=80; %encounter another leading vehicle 80m ahead with 70km/h
        end
        
    otherwise %% ******************************************* Leading Vehicle overspeed and move far away (CC-ACC)
        % t<9s leading car CC 60km/h ego car following
        % t=9s leading car accelerates with 2.5m/s^2 to 90km/h
        % ego car switch from ACC to CC at 80km/h
        if time<9
            v=60;
        else
            v=60+2.5*(time-9)*3.6;  %leading car 2.5m/s^2
            if v>90
                v=90;
            end
        end
        s0=60/3.6*td+2;%leading car initial location 
end

== matlab function ACC_CC_model_4_15/ACC-CC Switch ==
  data: d_logic1 output; d_logic2 output; u output; vset input; vp input; v input; d input; d_des input; lastmodel input
function [ d_logic1,d_logic2,u]  = fcn(vset,vp,v,d,d_des,lastmodel)
% u=1：ACC   U=2：CC
vset=vset/3.6;
vp=vp/3.6;
v=v/3.6;

k2=1.2;d1=2;
k1=1.999-1.196*exp(-0.1299*(vset-vp));
d_logic1=d_des+k1/2*(vset-vp)+k2*(v-vset)+d1;

k3=2;
d2=2;
k4=1.25;
d_logic2=d_des+k3*(vset-vp)+k4*(v-vp)+d2;

if vp>vset
    if d<d_des
        u=1;
    elseif (d>=d_des)&&(d<d_logic1)
        u=2;
    elseif (d>=d_logic1)&&(d<d_logic2)
        u=2;
    else
        u=2;
    end
else
    if d<d_des
        u=1;
    elseif (d>=d_des)&&(d<d_logic1)
        u=1;
    elseif (d>=d_logic1)&&(d<d_logic2)
        u=lastmodel;  %buffer
    else
        u=2;
    end
end
end
